simulink model "FunctionalArchitectureProj"  (R2023b)
settings: Solver=VariableStepAuto  StartTime=0.0  StopTime=10.0  RelTol=1e-3
(part 1 of 3)
settings Model: Creator=carol  LastModifiedBy=carol

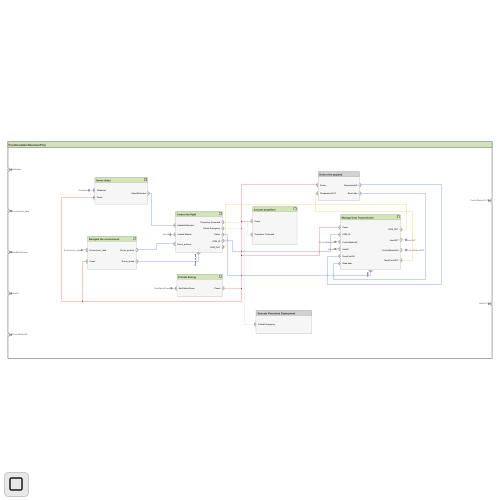
[thumbnail: Simulink's stored preview of the top-level diagram]
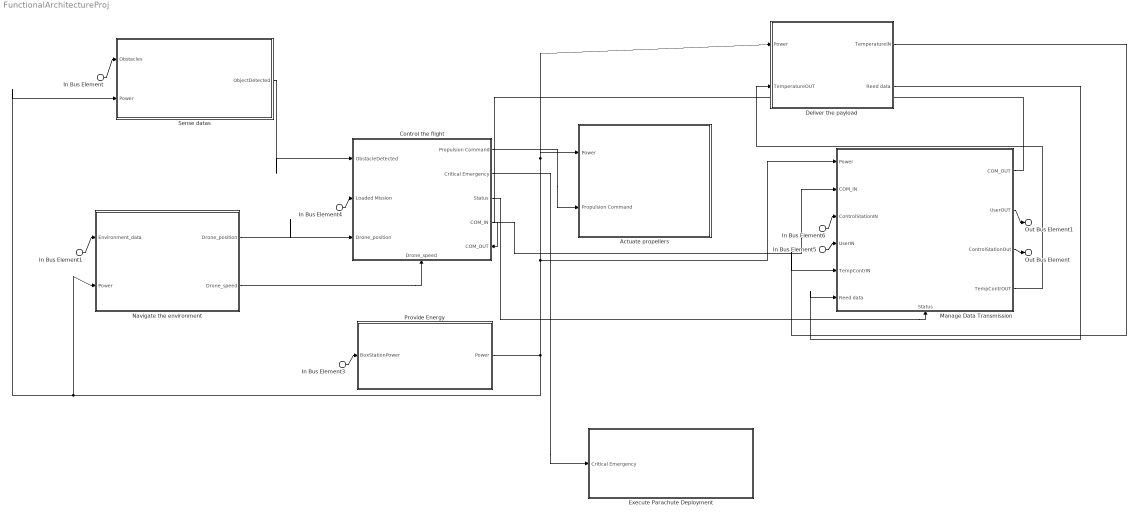
== system FunctionalArchitectureProj ==
  In Bus Element : Inport  PortName=Obstacles
  In Bus Element1 : Inport  Port=2  PortName=Environment_data
  In Bus Element3 : Inport  Port=3  PortName=BoxStationPower
  In Bus Element4 : Inport  Port=4  PortName=UserIN
  In Bus Element5 : Inport  Port=4  PortName=UserIN
  In Bus Element6 : Inport  Port=5  PortName=ControlStationIN
  " Execute Parachute Deployment" : Subsystem
      settings: PortSchema="{\"entries\":[{\"content\":{\"headerSize\":26,\"margin\":15,\"minimumSpacing\":25,\"sides\":[{\"content\":{\"connectorIds\":[\"In1\"]},\"type\":\"ConnectorPlacement.EquallySpacedRectSide\",\"uuid\":\"8049ad02-19ac-4f14-9b36-a42a8615a652\"},{\"content\":{\"side\":\"RIGHT\"},\"type\":\"ConnectorPlacement.EquallySpacedRectSide\",\"uuid\":\"a3e2e02d-3567-418c-afac-b08313eb92f4\"},{\"content\":{\"side\":\"TOP\"},\"type\":\"ConnectorPlacement.EquallySpacedRectSide\",\"uuid\":\"0a99e400-62af-4ce6-9b2a-3ec4b8645f60\"},{\"content\":{\"side\":\"BOTTOM\"},\"type\":\"ConnectorPlacement.EquallySpacedRectSide\",\"uuid\":\"e83c7a6e-944d-4583-b49e-8615a84d262f\"}]},\"type\":\"ConnectorPlacement.EquallySpacedConnector\",\"uuid\":\"ada0285e-d286-47a3-bd64-ce4f3c6c3017\"}],\"packageUris\":[\"http://schema.mathworks.com/mf0/Connector/R2020b\"],\"version\":\"1.0\"}"
  Actuate propellers : Subsystem
      settings: PortSchema="{\"entries\":[{\"content\":{\"headerSize\":26,\"margin\":15,\"minimumSpacing\":25,\"sides\":[{\"content\":{\"connectorIds\":[\"In1\",\"In2\"]},\"type\":\"ConnectorPlacement.EquallySpacedRectSide\",\"uuid\":\"9cca9539-0a36-4124-b22c-ee31f3591a67\"},{\"content\":{\"side\":\"RIGHT\"},\"type\":\"ConnectorPlacement.EquallySpacedRectSide\",\"uuid\":\"eebe1ec1-c849-468b-8863-53f0cc841d23\"},{\"content\":{\"side\":\"TOP\"},\"type\":\"ConnectorPlacement.EquallySpacedRectSide\",\"uuid\":\"8f1c4dda-9d7f-4fb5-99d0-4e96ed432329\"}]},\"type\":\"ConnectorPlacement.EquallySpacedConnector\",\"uuid\":\"f7d57f3a-667c-4dfa-8f30-8433699dfbc6\"}],\"packageUris\":[\"http://schema.mathworks.com/mf0/Connector/R2020b\"],\"version\":\"1.0\"}"
  Control the flight : Subsystem
      settings: PortSchema="{\"entries\":[{\"content\":{\"headerSize\":26,\"margin\":15,\"minimumSpacing\":25,\"sides\":[{\"content\":{\"connectorIds\":[\"In3\",\"In4\",\"In5\"]},\"type\":\"ConnectorPlacement.EquallySpacedRectSide\",\"uuid\":\"6ae6270c-bff4-4a0d-8fba-8fdec87b0a05\"},{\"content\":{\"connectorIds\":[\"Out1\",\"Out2\",\"Out3\",\"Out4\",\"In1\"],\"side\":\"RIGHT\"},\"type\":\"ConnectorPlacement.EquallySpacedRectSide\",\"uuid\":\"f3a0045b-bb3b-40f9-afd5-e1537ff3eeca\"},{\"content\":{\"side\":\"TOP\"},\"type\":\"ConnectorPlacement.EquallySpacedRectSide\",\"uuid\":\"e89a58f2-90b0-468c-bb6a-95617af68e24\"},{\"content\":{\"connectorIds\":[\"In2\"],\"side\":\"BOTTOM\"},\"type\":\"ConnectorPlacement.EquallySpacedRectSide\",\"uuid\":\"5f2fc7ae-0fcb-4b02-9512-f183f1206c8f\"}]},\"type\":\"ConnectorPlacement.EquallySpacedConnector\",\"uuid\":\"066eb43c-7b96-4660-9f29-628dd77a5b3b\"}],\"packageUris\":[\"http://schema.mathworks.com/mf0/Connector/R2020b\"],\"version\":\"1.0\"}"
  Deliver the payload : Subsystem
      settings: PortSchema="{\"entries\":[{\"content\":{\"headerSize\":26,\"margin\":15,\"minimumSpacing\":25,\"sides\":[{\"content\":{\"connectorIds\":[\"In1\",\"In2\"]},\"type\":\"ConnectorPlacement.EquallySpacedRectSide\",\"uuid\":\"8049ad02-19ac-4f14-9b36-a42a8615a652\"},{\"content\":{\"connectorIds\":[\"Out2\",\"Out1\"],\"side\":\"RIGHT\"},\"type\":\"ConnectorPlacement.EquallySpacedRectSide\",\"uuid\":\"a3e2e02d-3567-418c-afac-b08313eb92f4\"},{\"content\":{\"side\":\"TOP\"},\"type\":\"ConnectorPlacement.EquallySpacedRectSide\",\"uuid\":\"0a99e400-62af-4ce6-9b2a-3ec4b8645f60\"}]},\"type\":\"ConnectorPlacement.EquallySpacedConnector\",\"uuid\":\"ada0285e-d286-47a3-bd64-ce4f3c6c3017\"}],\"packageUris\":[\"http://schema.mathworks.com/mf0/Connector/R2020b\"],\"version\":\"1.0\"}"
  "Manage Data Transmission " : Subsystem
      settings: PortSchema="{\"entries\":[{\"content\":{\"headerSize\":26,\"margin\":15,\"minimumSpacing\":25,\"sides\":[{\"content\":{\"connectorIds\":[\"In2\",\"In3\",\"In4\",\"In5\",\"In7\",\"In6\"]},\"type\":\"ConnectorPlacement.EquallySpacedRectSide\",\"uuid\":\"9c17b9ef-2834-4c82-b9e5-e6d3fc257de6\"},{\"content\":{\"connectorIds\":[\"Out1\",\"Out2\",\"Out3\",\"Out4\"],\"side\":\"RIGHT\"},\"type\":\"ConnectorPlacement.EquallySpacedRectSide\",\"uuid\":\"9ecb8183-c057-4821-b5b4-2d9c431b5fb2\"},{\"content\":{\"side\":\"TOP\"},\"type\":\"ConnectorPlacement.EquallySpacedRectSide\",\"uuid\":\"bcbced7c-61ac-4e5d-8c11-0c5bb0f95d66\"},{\"content\":{\"connectorIds\":[\"In1\"],\"side\":\"BOTTOM\"},\"type\":\"ConnectorPlacement.EquallySpacedRectSide\",\"uuid\":\"08cd3b33-b135-4af9-aec5-206e0f2419c0\"}]},\"type\":\"ConnectorPlacement.EquallySpacedConnector\",\"uuid\":\"9e4a88fc-7b2c-4c70-8e8f-1bc090782de6\"}],\"packageUris\":[\"http://schema.mathworks.com/mf0/Connector/R2020b\"],\"version\":\"1.0\"}"
  Navigate the environment : Subsystem
      settings: PortSchema="{\"entries\":[{\"content\":{\"headerSize\":26,\"margin\":15,\"minimumSpacing\":25,\"sides\":[{\"content\":{\"connectorIds\":[\"In1\",\"In2\"]},\"type\":\"ConnectorPlacement.EquallySpacedRectSide\",\"uuid\":\"3b5ec35b-efef-42bc-989f-0358b373f88c\"},{\"content\":{\"connectorIds\":[\"Out1\",\"Out2\"],\"side\":\"RIGHT\"},\"type\":\"ConnectorPlacement.EquallySpacedRectSide\",\"uuid\":\"39a24d49-19b9-4508-91cd-8aceba2ac1ea\"},{\"content\":{\"side\":\"TOP\"},\"type\":\"ConnectorPlacement.EquallySpacedRectSide\",\"uuid\":\"1edcc8ed-84b2-4c5f-810f-53183898c4f5\"}]},\"type\":\"ConnectorPlacement.EquallySpacedConnector\",\"uuid\":\"9d581d8a-2dea-49e6-903e-7a6990d5505f\"}],\"packageUris\":[\"http://schema.mathworks.com/mf0/Connector/R2020b\"],\"version\":\"1.0\"}"
  Provide Energy : Subsystem
      settings: PortSchema="{\"entries\":[{\"content\":{\"headerSize\":26,\"margin\":15,\"minimumSpacing\":25,\"sides\":[{\"content\":{\"connectorIds\":[\"In1\"]},\"type\":\"ConnectorPlacement.EquallySpacedRectSide\",\"uuid\":\"6ae6270c-bff4-4a0d-8fba-8fdec87b0a05\"},{\"content\":{\"connectorIds\":[\"Out1\"],\"side\":\"RIGHT\"},\"type\":\"ConnectorPlacement.EquallySpacedRectSide\",\"uuid\":\"f3a0045b-bb3b-40f9-afd5-e1537ff3eeca\"},{\"content\":{\"side\":\"TOP\"},\"type\":\"ConnectorPlacement.EquallySpacedRectSide\",\"uuid\":\"e89a58f2-90b0-468c-bb6a-95617af68e24\"}]},\"type\":\"ConnectorPlacement.EquallySpacedConnector\",\"uuid\":\"066eb43c-7b96-4660-9f29-628dd77a5b3b\"}],\"packageUris\":[\"http://schema.mathworks.com/mf0/Connector/R2020b\"],\"version\":\"1.0\"}"
  Sense datas : Subsystem
      settings: PortSchema="{\"entries\":[{\"content\":{\"headerSize\":26,\"margin\":15,\"minimumSpacing\":25,\"sides\":[{\"content\":{\"connectorIds\":[\"In1\",\"In2\"]},\"type\":\"ConnectorPlacement.EquallySpacedRectSide\",\"uuid\":\"6ae6270c-bff4-4a0d-8fba-8fdec87b0a05\"},{\"content\":{\"connectorIds\":[\"Out1\"],\"side\":\"RIGHT\"},\"type\":\"ConnectorPlacement.EquallySpacedRectSide\",\"uuid\":\"f3a0045b-bb3b-40f9-afd5-e1537ff3eeca\"},{\"content\":{\"side\":\"TOP\"},\"type\":\"ConnectorPlacement.EquallySpacedRectSide\",\"uuid\":\"e89a58f2-90b0-468c-bb6a-95617af68e24\"}]},\"type\":\"ConnectorPlacement.EquallySpacedConnector\",\"uuid\":\"066eb43c-7b96-4660-9f29-628dd77a5b3b\"}],\"packageUris\":[\"http://schema.mathworks.com/mf0/Connector/R2020b\"],\"version\":\"1.0\"}"
  Out Bus Element : Outport  PortName=ControlStationOUT
  Out Bus Element1 : Outport  Port=2  PortName=UserOUT
  wires:
  In Bus Element3/1 -> Provide Energy/1(BoxStationPower)
  In Bus Element1/1 -> Navigate the environment/1(Environment_data)
  In Bus Element/1 -> Sense datas/1(Obstacles)
  Control the flight/1(Propulsion Command) -> Actuate propellers/2(Propulsion Command)
  Sense datas/1(ObjectDetected) -> Control the flight/3(ObstacleDetected)
  Navigate the environment/1(Drone_position) -> Control the flight/5(Drone_position)
  Navigate the environment/2(Drone_speed) -> Control the flight/2(Drone_speed)
  Provide Energy/1(Power) -> Navigate the environment/2(Power), Sense datas/2(Power), "Manage Data Transmission "/2(Power), Deliver the payload/1(Power), Actuate propellers/1(Power)
  Control the flight/2(Critical Emergency) -> " Execute Parachute Deployment"/1(Critical Emergency)
  Control the flight/3(Status) -> "Manage Data Transmission "/1(Status)
  Control the flight/4(COM_IN) -> "Manage Data Transmission "/3(COM_IN)
  "Manage Data Transmission "/1(COM_OUT) -> Control the flight/1(COM_OUT)
  In Bus Element4/1 -> Control the flight/4(Loaded Mission)
  In Bus Element5/1 -> "Manage Data Transmission "/5(UserIN)
  "Manage Data Transmission "/2(UserOUT) -> Out Bus Element1/1
  "Manage Data Transmission "/3(ControlStationOut) -> Out Bus Element/1
  "Manage Data Transmission "/4(TempContrOUT) -> Deliver the payload/2(TemperatureOUT)
  Deliver the payload/2(TemperatureIN) -> "Manage Data Transmission "/7(TempContrIN)
  Deliver the payload/1(Reed data) -> "Manage Data Transmission "/6(Reed data)
  In Bus Element6/1 -> "Manage Data Transmission "/4(ControlStationIN)

== system FunctionalArchitectureProj/ Execute Parachute Deployment ==
  Bus Element In1 : Inport  PortName=Critical Emergency
  Detect emergency : Subsystem
      settings: PortSchema="{\"entries\":[{\"content\":{\"headerSize\":26,\"margin\":15,\"minimumSpacing\":25,\"sides\":[{\"content\":{\"connectorIds\":[\"In1\"]},\"type\":\"ConnectorPlacement.EquallySpacedRectSide\",\"uuid\":\"8049ad02-19ac-4f14-9b36-a42a8615a652\"},{\"content\":{\"connectorIds\":[\"Out1\"],\"side\":\"RIGHT\"},\"type\":\"ConnectorPlacement.EquallySpacedRectSide\",\"uuid\":\"a3e2e02d-3567-418c-afac-b08313eb92f4\"},{\"content\":{\"side\":\"TOP\"},\"type\":\"ConnectorPlacement.EquallySpacedRectSide\",\"uuid\":\"0a99e400-62af-4ce6-9b2a-3ec4b8645f60\"}]},\"type\":\"ConnectorPlacement.EquallySpacedConnector\",\"uuid\":\"ada0285e-d286-47a3-bd64-ce4f3c6c3017\"}],\"packageUris\":[\"http://schema.mathworks.com/mf0/Connector/R2020b\"],\"version\":\"1.0\"}"
  Execute the parachute : Subsystem
      settings: PortSchema="{\"entries\":[{\"content\":{\"headerSize\":26,\"margin\":15,\"minimumSpacing\":25,\"sides\":[{\"content\":{\"connectorIds\":[\"In1\"]},\"type\":\"ConnectorPlacement.EquallySpacedRectSide\",\"uuid\":\"8049ad02-19ac-4f14-9b36-a42a8615a652\"},{\"content\":{\"side\":\"RIGHT\"},\"type\":\"ConnectorPlacement.EquallySpacedRectSide\",\"uuid\":\"a3e2e02d-3567-418c-afac-b08313eb92f4\"},{\"content\":{\"side\":\"TOP\"},\"type\":\"ConnectorPlacement.EquallySpacedRectSide\",\"uuid\":\"0a99e400-62af-4ce6-9b2a-3ec4b8645f60\"}]},\"type\":\"ConnectorPlacement.EquallySpacedConnector\",\"uuid\":\"ada0285e-d286-47a3-bd64-ce4f3c6c3017\"}],\"packageUris\":[\"http://schema.mathworks.com/mf0/Connector/R2020b\"],\"version\":\"1.0\"}"
  Trigger the mechanism : Subsystem
      settings: PortSchema="{\"entries\":[{\"content\":{\"headerSize\":26,\"margin\":15,\"minimumSpacing\":25,\"sides\":[{\"content\":{\"connectorIds\":[\"In1\"]},\"type\":\"ConnectorPlacement.EquallySpacedRectSide\",\"uuid\":\"8049ad02-19ac-4f14-9b36-a42a8615a652\"},{\"content\":{\"connectorIds\":[\"Out1\"],\"side\":\"RIGHT\"},\"type\":\"ConnectorPlacement.EquallySpacedRectSide\",\"uuid\":\"a3e2e02d-3567-418c-afac-b08313eb92f4\"},{\"content\":{\"side\":\"TOP\"},\"type\":\"ConnectorPlacement.EquallySpacedRectSide\",\"uuid\":\"0a99e400-62af-4ce6-9b2a-3ec4b8645f60\"}]},\"type\":\"ConnectorPlacement.EquallySpacedConnector\",\"uuid\":\"ada0285e-d286-47a3-bd64-ce4f3c6c3017\"}],\"packageUris\":[\"http://schema.mathworks.com/mf0/Connector/R2020b\"],\"version\":\"1.0\"}"
  wires:
  Detect emergency/1(alert_signal) -> Trigger the mechanism/1(alert_signal)
  Trigger the mechanism/1(Trigger _signal) -> Execute the parachute/1(Trigger _signal)
  Bus Element In1/1 -> Detect emergency/1(Critical Emergency)

== system FunctionalArchitectureProj/Actuate propellers ==
  Bus Element In1 : Inport  PortName=Power
  Bus Element In6 : Inport  Port=2  PortName=Propulsion Command
  Regulate speed of Propeller : Subsystem
      settings: PortSchema="{\"entries\":[{\"content\":{\"headerSize\":26,\"margin\":15,\"minimumSpacing\":25,\"sides\":[{\"content\":{\"connectorIds\":[\"In2\"]},\"type\":\"ConnectorPlacement.EquallySpacedRectSide\",\"uuid\":\"c0b5e0bb-d2bf-4d40-b1ad-0d63f5f2311e\"},{\"content\":{\"connectorIds\":[\"Out1\"],\"side\":\"RIGHT\"},\"type\":\"ConnectorPlacement.EquallySpacedRectSide\",\"uuid\":\"73104a81-7012-49ca-8030-68cbb7243dfa\"},{\"content\":{\"side\":\"TOP\"},\"type\":\"ConnectorPlacement.EquallySpacedRectSide\",\"uuid\":\"7c311739-eaa1-403c-a576-4458554363b2\"},{\"content\":{\"connectorIds\":[\"In1\"],\"side\":\"BOTTOM\"},\"type\":\"ConnectorPlacement.EquallySpacedRectSide\",\"uuid\":\"afa3ef7d-980f-4119-97e5-3dc0677e5f7e\"}]},\"type\":\"ConnectorPlacement.EquallySpacedConnector\",\"uuid\":\"83a80a93-0958-4176-98e5-b02d609066aa\"}],\"packageUris\":[\"http://schema.mathworks.com/mf0/Connector/R2020b\"],\"version\":\"1.0\"}"
  Set Target speed of propellers : Subsystem
      settings: PortSchema="{\"entries\":[{\"content\":{\"headerSize\":26,\"margin\":15,\"minimumSpacing\":25,\"sides\":[{\"content\":{\"connectorIds\":[\"In1\"]},\"type\":\"ConnectorPlacement.EquallySpacedRectSide\",\"uuid\":\"c0b5e0bb-d2bf-4d40-b1ad-0d63f5f2311e\"},{\"content\":{\"connectorIds\":[\"Out1\"],\"side\":\"RIGHT\"},\"type\":\"ConnectorPlacement.EquallySpacedRectSide\",\"uuid\":\"73104a81-7012-49ca-8030-68cbb7243dfa\"},{\"content\":{\"side\":\"TOP\"},\"type\":\"ConnectorPlacement.EquallySpacedRectSide\",\"uuid\":\"7c311739-eaa1-403c-a576-4458554363b2\"}]},\"type\":\"ConnectorPlacement.EquallySpacedConnector\",\"uuid\":\"83a80a93-0958-4176-98e5-b02d609066aa\"}],\"packageUris\":[\"http://schema.mathworks.com/mf0/Connector/R2020b\"],\"version\":\"1.0\"}"
  Split the energy : Subsystem
      settings: PortSchema="{\"entries\":[{\"content\":{\"headerSize\":26,\"margin\":15,\"minimumSpacing\":25,\"sides\":[{\"content\":{\"connectorIds\":[\"In1\",\"In2\"]},\"type\":\"ConnectorPlacement.EquallySpacedRectSide\",\"uuid\":\"c0b5e0bb-d2bf-4d40-b1ad-0d63f5f2311e\"},{\"content\":{\"connectorIds\":[\"Out1\"],\"side\":\"RIGHT\"},\"type\":\"ConnectorPlacement.EquallySpacedRectSide\",\"uuid\":\"73104a81-7012-49ca-8030-68cbb7243dfa\"},{\"content\":{\"connectorIds\":[],\"side\":\"TOP\"},\"type\":\"ConnectorPlacement.EquallySpacedRectSide\",\"uuid\":\"7c311739-eaa1-403c-a576-4458554363b2\"},{\"content\":{\"connectorIds\":[],\"side\":\"BOTTOM\"},\"type\":\"ConnectorPlacement.EquallySpacedRectSide\",\"uuid\":\"ef70e0e5-7c28-4d60-a2ab-1af0db1b5348\"}]},\"type\":\"ConnectorPlacement.EquallySpacedConnector\",\"uuid\":\"83a80a93-0958-4176-98e5-b02d609066aa\"}],\"packageUris\":[\"http://schema.mathworks.com/mf0/Connector/R2020b\"],\"version\":\"1.0\"}"
  wires:
  Bus Element In6/1 -> Set Target speed of propellers/1(Propulsion Command)
  Set Target speed of propellers/1(Target_Speed) -> Regulate speed of Propeller/2(Target_Speed)
  Regulate speed of Propeller/1(data) -> Split the energy/2(data)
  Split the energy/1(Single Motor Voltage) -> Regulate speed of Propeller/1(Single Motor Voltage)
  Bus Element In1/1 -> Split the energy/1(Power)

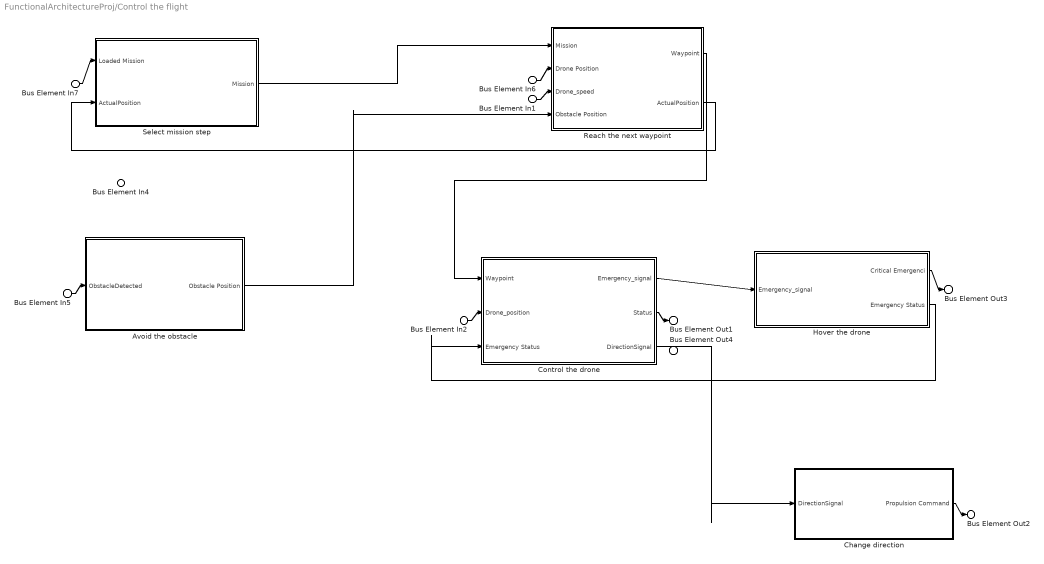
== system FunctionalArchitectureProj/Control the flight ==
  Bus Element In4 : Inport  PortName=COM_OUT
  Bus Element In1 : Inport  Port=2  PortName=Drone_speed
  Bus Element In5 : Inport  Port=3  PortName=ObstacleDetected
  Bus Element In7 : Inport  Port=4  PortName=Loaded Mission
  Bus Element In6 : Inport  Port=5  PortName=Drone_position
  Bus Element In2 : Inport  Port=5  PortName=Drone_position
  Avoid the obstacle : Subsystem
      settings: PortSchema="{\"entries\":[{\"content\":{\"headerSize\":26,\"margin\":15,\"minimumSpacing\":25,\"sides\":[{\"content\":{\"connectorIds\":[\"In1\"]},\"type\":\"ConnectorPlacement.EquallySpacedRectSide\",\"uuid\":\"9cca9539-0a36-4124-b22c-ee31f3591a67\"},{\"content\":{\"connectorIds\":[\"Out1\"],\"side\":\"RIGHT\"},\"type\":\"ConnectorPlacement.EquallySpacedRectSide\",\"uuid\":\"eebe1ec1-c849-468b-8863-53f0cc841d23\"},{\"content\":{\"connectorIds\":[],\"side\":\"TOP\"},\"type\":\"ConnectorPlacement.EquallySpacedRectSide\",\"uuid\":\"8f1c4dda-9d7f-4fb5-99d0-4e96ed432329\"}]},\"type\":\"ConnectorPlacement.EquallySpacedConnector\",\"uuid\":\"f7d57f3a-667c-4dfa-8f30-8433699dfbc6\"}],\"packageUris\":[\"http://schema.mathworks.com/mf0/Connector/R2020b\"],\"version\":\"1.0\"}"
  Change direction : Subsystem
      settings: PortSchema="{\"entries\":[{\"content\":{\"headerSize\":26,\"margin\":15,\"minimumSpacing\":25,\"sides\":[{\"content\":{\"connectorIds\":[\"In1\"]},\"type\":\"ConnectorPlacement.EquallySpacedRectSide\",\"uuid\":\"9cca9539-0a36-4124-b22c-ee31f3591a67\"},{\"content\":{\"connectorIds\":[\"Out1\"],\"side\":\"RIGHT\"},\"type\":\"ConnectorPlacement.EquallySpacedRectSide\",\"uuid\":\"eebe1ec1-c849-468b-8863-53f0cc841d23\"},{\"content\":{\"side\":\"TOP\"},\"type\":\"ConnectorPlacement.EquallySpacedRectSide\",\"uuid\":\"8f1c4dda-9d7f-4fb5-99d0-4e96ed432329\"}]},\"type\":\"ConnectorPlacement.EquallySpacedConnector\",\"uuid\":\"f7d57f3a-667c-4dfa-8f30-8433699dfbc6\"}],\"packageUris\":[\"http://schema.mathworks.com/mf0/Connector/R2020b\"],\"version\":\"1.0\"}"
  Control the drone : Subsystem
      settings: PortSchema="{\"entries\":[{\"content\":{\"headerSize\":26,\"margin\":15,\"minimumSpacing\":25,\"sides\":[{\"content\":{\"connectorIds\":[\"In1\",\"In2\",\"In3\"]},\"type\":\"ConnectorPlacement.EquallySpacedRectSide\",\"uuid\":\"ae43e0f9-cb81-4c7d-a5a1-6ddd261c3f36\"},{\"content\":{\"connectorIds\":[\"Out1\",\"Out2\",\"Out3\"],\"side\":\"RIGHT\"},\"type\":\"ConnectorPlacement.EquallySpacedRectSide\",\"uuid\":\"454013ea-826f-4879-bd33-a0fc10a3e69e\"},{\"content\":{\"connectorIds\":[],\"side\":\"TOP\"},\"type\":\"ConnectorPlacement.EquallySpacedRectSide\",\"uuid\":\"d045879a-9dfe-4c38-a274-6118b00e003b\"}]},\"type\":\"ConnectorPlacement.EquallySpacedConnector\",\"uuid\":\"e33c714e-0ae2-4a56-8ce0-f9b8de85daa2\"}],\"packageUris\":[\"http://schema.mathworks.com/mf0/Connector/R2020b\"],\"version\":\"1.0\"}"
  Hover the drone : Subsystem
      settings: PortSchema="{\"entries\":[{\"content\":{\"headerSize\":26,\"margin\":15,\"minimumSpacing\":25,\"sides\":[{\"content\":{\"connectorIds\":[\"In1\"]},\"type\":\"ConnectorPlacement.EquallySpacedRectSide\",\"uuid\":\"ae43e0f9-cb81-4c7d-a5a1-6ddd261c3f36\"},{\"content\":{\"connectorIds\":[\"Out1\",\"Out2\"],\"side\":\"RIGHT\"},\"type\":\"ConnectorPlacement.EquallySpacedRectSide\",\"uuid\":\"454013ea-826f-4879-bd33-a0fc10a3e69e\"},{\"content\":{\"connectorIds\":[],\"side\":\"TOP\"},\"type\":\"ConnectorPlacement.EquallySpacedRectSide\",\"uuid\":\"d045879a-9dfe-4c38-a274-6118b00e003b\"}]},\"type\":\"ConnectorPlacement.EquallySpacedConnector\",\"uuid\":\"e33c714e-0ae2-4a56-8ce0-f9b8de85daa2\"}],\"packageUris\":[\"http://schema.mathworks.com/mf0/Connector/R2020b\"],\"version\":\"1.0\"}"
  Reach the next waypoint : Subsystem
      settings: PortSchema="{\"entries\":[{\"content\":{\"headerSize\":26,\"margin\":15,\"minimumSpacing\":25,\"sides\":[{\"content\":{\"connectorIds\":[\"In1\",\"In2\",\"In3\",\"In4\"]},\"type\":\"ConnectorPlacement.EquallySpacedRectSide\",\"uuid\":\"ae43e0f9-cb81-4c7d-a5a1-6ddd261c3f36\"},{\"content\":{\"connectorIds\":[\"Out2\",\"Out1\"],\"side\":\"RIGHT\"},\"type\":\"ConnectorPlacement.EquallySpacedRectSide\",\"uuid\":\"454013ea-826f-4879-bd33-a0fc10a3e69e\"},{\"content\":{\"connectorIds\":[],\"side\":\"TOP\"},\"type\":\"ConnectorPlacement.EquallySpacedRectSide\",\"uuid\":\"d045879a-9dfe-4c38-a274-6118b00e003b\"}]},\"type\":\"ConnectorPlacement.EquallySpacedConnector\",\"uuid\":\"e33c714e-0ae2-4a56-8ce0-f9b8de85daa2\"}],\"packageUris\":[\"http://schema.mathworks.com/mf0/Connector/R2020b\"],\"version\":\"1.0\"}"
  Select mission step : Subsystem
      settings: PortSchema="{\"entries\":[{\"content\":{\"headerSize\":26,\"margin\":15,\"minimumSpacing\":25,\"sides\":[{\"content\":{\"connectorIds\":[\"In1\",\"In2\"]},\"type\":\"ConnectorPlacement.EquallySpacedRectSide\",\"uuid\":\"ae43e0f9-cb81-4c7d-a5a1-6ddd261c3f36\"},{\"content\":{\"connectorIds\":[\"Out1\"],\"side\":\"RIGHT\"},\"type\":\"ConnectorPlacement.EquallySpacedRectSide\",\"uuid\":\"454013ea-826f-4879-bd33-a0fc10a3e69e\"},{\"content\":{\"connectorIds\":[],\"side\":\"TOP\"},\"type\":\"ConnectorPlacement.EquallySpacedRectSide\",\"uuid\":\"d045879a-9dfe-4c38-a274-6118b00e003b\"}]},\"type\":\"ConnectorPlacement.EquallySpacedConnector\",\"uuid\":\"e33c714e-0ae2-4a56-8ce0-f9b8de85daa2\"}],\"packageUris\":[\"http://schema.mathworks.com/mf0/Connector/R2020b\"],\"version\":\"1.0\"}"
  Bus Element Out2 : Outport  PortName=Propulsion Command
  Bus Element Out3 : Outport  Port=2  PortName=Critical Emergency
  Bus Element Out1 : Outport  Port=3  PortName=Status
  Bus Element Out4 : Outport  Port=4  PortName=COM_IN
  wires:
  Bus Element In5/1 -> Avoid the obstacle/1(ObstacleDetected)
  Bus Element In6/1 -> Reach the next waypoint/2(Drone Position)
  Select mission step/1(Mission) -> Reach the next waypoint/1(Mission)
  Reach the next waypoint/1(ActualPosition) -> Select mission step/2(ActualPosition)
  Bus Element In7/1 -> Select mission step/1(Loaded Mission)
  Change direction/1(Propulsion Command) -> Bus Element Out2/1
  Bus Element In1/1 -> Reach the next waypoint/3(Drone_speed)
  Control the drone/2(Status) -> Bus Element Out1/1
  Avoid the obstacle/1(Obstacle Position) -> Reach the next waypoint/4(Obstacle Position)
  Reach the next waypoint/2(Waypoint) -> Control the drone/1(Waypoint)
  Control the drone/3(DirectionSignal) -> Change direction/1(DirectionSignal)
  Bus Element In2/1 -> Control the drone/2(Drone_position)
  Control the drone/1(Emergency_signal) -> Hover the drone/1(Emergency_signal)
  Hover the drone/1(Critical Emergenci) -> Bus Element Out3/1
  Hover the drone/2(Emergency Status) -> Control the drone/3(Emergency Status)

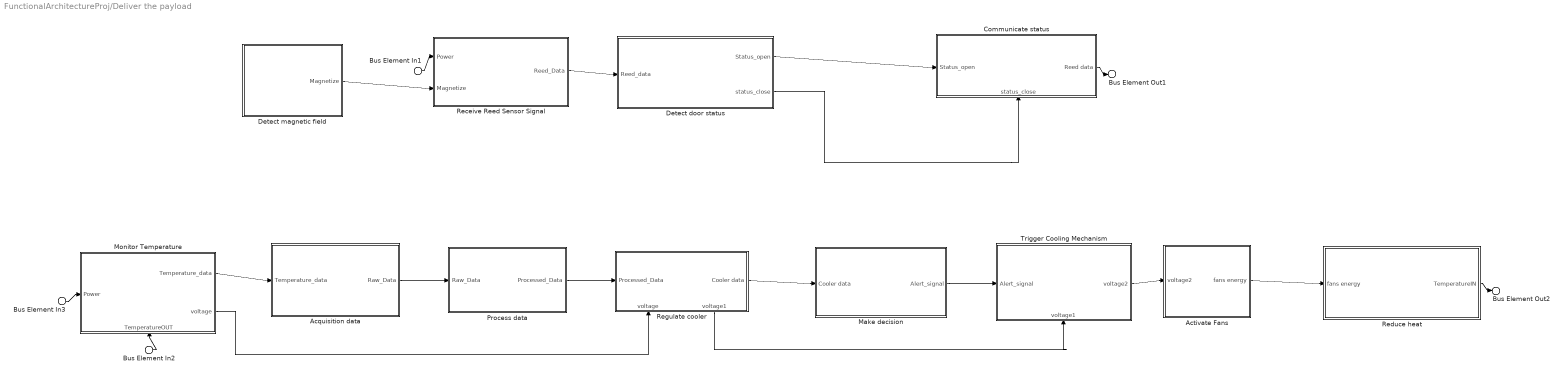
== system FunctionalArchitectureProj/Deliver the payload ==
  Bus Element In1 : Inport  PortName=Power
  Bus Element In3 : Inport  PortName=Power
  Bus Element In2 : Inport  Port=2  PortName=TemperatureOUT
  Acquisition data : Subsystem
      settings: PortSchema="{\"entries\":[{\"content\":{\"headerSize\":26,\"margin\":15,\"minimumSpacing\":25,\"sides\":[{\"content\":{\"connectorIds\":[\"In1\"]},\"type\":\"ConnectorPlacement.EquallySpacedRectSide\",\"uuid\":\"8049ad02-19ac-4f14-9b36-a42a8615a652\"},{\"content\":{\"connectorIds\":[\"Out1\"],\"side\":\"RIGHT\"},\"type\":\"ConnectorPlacement.EquallySpacedRectSide\",\"uuid\":\"a3e2e02d-3567-418c-afac-b08313eb92f4\"},{\"content\":{\"side\":\"TOP\"},\"type\":\"ConnectorPlacement.EquallySpacedRectSide\",\"uuid\":\"0a99e400-62af-4ce6-9b2a-3ec4b8645f60\"}]},\"type\":\"ConnectorPlacement.EquallySpacedConnector\",\"uuid\":\"ada0285e-d286-47a3-bd64-ce4f3c6c3017\"}],\"packageUris\":[\"http://schema.mathworks.com/mf0/Connector/R2020b\"],\"version\":\"1.0\"}"
  Activate Fans : Subsystem
      settings: PortSchema="{\"entries\":[{\"content\":{\"headerSize\":26,\"margin\":15,\"minimumSpacing\":25,\"sides\":[{\"content\":{\"connectorIds\":[\"In1\"]},\"type\":\"ConnectorPlacement.EquallySpacedRectSide\",\"uuid\":\"54e1fb7b-9e45-462f-884a-02984b69df8e\"},{\"content\":{\"connectorIds\":[\"Out1\"],\"side\":\"RIGHT\"},\"type\":\"ConnectorPlacement.EquallySpacedRectSide\",\"uuid\":\"bc959cb6-5763-4613-9c0f-216dfc1c8721\"},{\"content\":{\"side\":\"TOP\"},\"type\":\"ConnectorPlacement.EquallySpacedRectSide\",\"uuid\":\"3094b2e1-2656-4eb0-a370-e33613cb9a3e\"}]},\"type\":\"ConnectorPlacement.EquallySpacedConnector\",\"uuid\":\"4e036095-9cf9-4f63-b3c0-cf00d09848ce\"}],\"packageUris\":[\"http://schema.mathworks.com/mf0/Connector/R2020b\"],\"version\":\"1.0\"}"
  Communicate status : Subsystem
      settings: PortSchema="{\"entries\":[{\"content\":{\"headerSize\":26,\"margin\":15,\"minimumSpacing\":25,\"sides\":[{\"content\":{\"connectorIds\":[\"In1\"]},\"type\":\"ConnectorPlacement.EquallySpacedRectSide\",\"uuid\":\"8049ad02-19ac-4f14-9b36-a42a8615a652\"},{\"content\":{\"connectorIds\":[\"Out1\"],\"side\":\"RIGHT\"},\"type\":\"ConnectorPlacement.EquallySpacedRectSide\",\"uuid\":\"a3e2e02d-3567-418c-afac-b08313eb92f4\"},{\"content\":{\"side\":\"TOP\"},\"type\":\"ConnectorPlacement.EquallySpacedRectSide\",\"uuid\":\"0a99e400-62af-4ce6-9b2a-3ec4b8645f60\"},{\"content\":{\"connectorIds\":[\"In2\"],\"side\":\"BOTTOM\"},\"type\":\"ConnectorPlacement.EquallySpacedRectSide\",\"uuid\":\"af5b728c-4ca3-4e93-bc61-3fa3a4a27f8e\"}]},\"type\":\"ConnectorPlacement.EquallySpacedConnector\",\"uuid\":\"ada0285e-d286-47a3-bd64-ce4f3c6c3017\"}],\"packageUris\":[\"http://schema.mathworks.com/mf0/Connector/R2020b\"],\"version\":\"1.0\"}"
  Detect door status : Subsystem
      settings: PortSchema="{\"entries\":[{\"content\":{\"headerSize\":26,\"margin\":15,\"minimumSpacing\":25,\"sides\":[{\"content\":{\"connectorIds\":[\"In1\"]},\"type\":\"ConnectorPlacement.EquallySpacedRectSide\",\"uuid\":\"8049ad02-19ac-4f14-9b36-a42a8615a652\"},{\"content\":{\"connectorIds\":[\"Out1\",\"Out2\"],\"side\":\"RIGHT\"},\"type\":\"ConnectorPlacement.EquallySpacedRectSide\",\"uuid\":\"a3e2e02d-3567-418c-afac-b08313eb92f4\"},{\"content\":{\"side\":\"TOP\"},\"type\":\"ConnectorPlacement.EquallySpacedRectSide\",\"uuid\":\"0a99e400-62af-4ce6-9b2a-3ec4b8645f60\"}]},\"type\":\"ConnectorPlacement.EquallySpacedConnector\",\"uuid\":\"ada0285e-d286-47a3-bd64-ce4f3c6c3017\"}],\"packageUris\":[\"http://schema.mathworks.com/mf0/Connector/R2020b\"],\"version\":\"1.0\"}"
  Detect magnetic field : Subsystem
      settings: PortSchema="{\"entries\":[{\"content\":{\"headerSize\":26,\"margin\":15,\"minimumSpacing\":25,\"sides\":[{\"content\":{},\"type\":\"ConnectorPlacement.EquallySpacedRectSide\",\"uuid\":\"8049ad02-19ac-4f14-9b36-a42a8615a652\"},{\"content\":{\"connectorIds\":[\"Out1\"],\"side\":\"RIGHT\"},\"type\":\"ConnectorPlacement.EquallySpacedRectSide\",\"uuid\":\"a3e2e02d-3567-418c-afac-b08313eb92f4\"},{\"content\":{\"side\":\"TOP\"},\"type\":\"ConnectorPlacement.EquallySpacedRectSide\",\"uuid\":\"0a99e400-62af-4ce6-9b2a-3ec4b8645f60\"}]},\"type\":\"ConnectorPlacement.EquallySpacedConnector\",\"uuid\":\"ada0285e-d286-47a3-bd64-ce4f3c6c3017\"}],\"packageUris\":[\"http://schema.mathworks.com/mf0/Connector/R2020b\"],\"version\":\"1.0\"}"
  Make decision : Subsystem
      settings: PortSchema="{\"entries\":[{\"content\":{\"headerSize\":26,\"margin\":15,\"minimumSpacing\":25,\"sides\":[{\"content\":{\"connectorIds\":[\"In1\"]},\"type\":\"ConnectorPlacement.EquallySpacedRectSide\",\"uuid\":\"8049ad02-19ac-4f14-9b36-a42a8615a652\"},{\"content\":{\"connectorIds\":[\"Out1\"],\"side\":\"RIGHT\"},\"type\":\"ConnectorPlacement.EquallySpacedRectSide\",\"uuid\":\"a3e2e02d-3567-418c-afac-b08313eb92f4\"},{\"content\":{\"side\":\"TOP\"},\"type\":\"ConnectorPlacement.EquallySpacedRectSide\",\"uuid\":\"0a99e400-62af-4ce6-9b2a-3ec4b8645f60\"}]},\"type\":\"ConnectorPlacement.EquallySpacedConnector\",\"uuid\":\"ada0285e-d286-47a3-bd64-ce4f3c6c3017\"}],\"packageUris\":[\"http://schema.mathworks.com/mf0/Connector/R2020b\"],\"version\":\"1.0\"}"
  "Monitor Temperature " : Subsystem
      settings: PortSchema="{\"entries\":[{\"content\":{\"headerSize\":26,\"margin\":15,\"minimumSpacing\":25,\"sides\":[{\"content\":{\"connectorIds\":[\"In2\"]},\"type\":\"ConnectorPlacement.EquallySpacedRectSide\",\"uuid\":\"8049ad02-19ac-4f14-9b36-a42a8615a652\"},{\"content\":{\"connectorIds\":[\"Out1\",\"Out2\"],\"side\":\"RIGHT\"},\"type\":\"ConnectorPlacement.EquallySpacedRectSide\",\"uuid\":\"a3e2e02d-3567-418c-afac-b08313eb92f4\"},{\"content\":{\"side\":\"TOP\"},\"type\":\"ConnectorPlacement.EquallySpacedRectSide\",\"uuid\":\"0a99e400-62af-4ce6-9b2a-3ec4b8645f60\"},{\"content\":{\"connectorIds\":[\"In1\"],\"side\":\"BOTTOM\"},\"type\":\"ConnectorPlacement.EquallySpacedRectSide\",\"uuid\":\"3dac5849-8858-4d39-ad28-a0a278f58204\"}]},\"type\":\"ConnectorPlacement.EquallySpacedConnector\",\"uuid\":\"ada0285e-d286-47a3-bd64-ce4f3c6c3017\"}],\"packageUris\":[\"http://schema.mathworks.com/mf0/Connector/R2020b\"],\"version\":\"1.0\"}"
  Process data : Subsystem
      settings: PortSchema="{\"entries\":[{\"content\":{\"headerSize\":26,\"margin\":15,\"minimumSpacing\":25,\"sides\":[{\"content\":{\"connectorIds\":[\"In1\"]},\"type\":\"ConnectorPlacement.EquallySpacedRectSide\",\"uuid\":\"8049ad02-19ac-4f14-9b36-a42a8615a652\"},{\"content\":{\"connectorIds\":[\"Out1\"],\"side\":\"RIGHT\"},\"type\":\"ConnectorPlacement.EquallySpacedRectSide\",\"uuid\":\"a3e2e02d-3567-418c-afac-b08313eb92f4\"},{\"content\":{\"side\":\"TOP\"},\"type\":\"ConnectorPlacement.EquallySpacedRectSide\",\"uuid\":\"0a99e400-62af-4ce6-9b2a-3ec4b8645f60\"}]},\"type\":\"ConnectorPlacement.EquallySpacedConnector\",\"uuid\":\"ada0285e-d286-47a3-bd64-ce4f3c6c3017\"}],\"packageUris\":[\"http://schema.mathworks.com/mf0/Connector/R2020b\"],\"version\":\"1.0\"}"
  Receive Reed Sensor Signal : Subsystem
      settings: PortSchema="{\"entries\":[{\"content\":{\"headerSize\":26,\"margin\":15,\"minimumSpacing\":25,\"sides\":[{\"content\":{\"connectorIds\":[\"In1\",\"In2\"]},\"type\":\"ConnectorPlacement.EquallySpacedRectSide\",\"uuid\":\"8049ad02-19ac-4f14-9b36-a42a8615a652\"},{\"content\":{\"connectorIds\":[\"Out1\"],\"side\":\"RIGHT\"},\"type\":\"ConnectorPlacement.EquallySpacedRectSide\",\"uuid\":\"a3e2e02d-3567-418c-afac-b08313eb92f4\"},{\"content\":{\"side\":\"TOP\"},\"type\":\"ConnectorPlacement.EquallySpacedRectSide\",\"uuid\":\"0a99e400-62af-4ce6-9b2a-3ec4b8645f60\"}]},\"type\":\"ConnectorPlacement.EquallySpacedConnector\",\"uuid\":\"ada0285e-d286-47a3-bd64-ce4f3c6c3017\"}],\"packageUris\":[\"http://schema.mathworks.com/mf0/Connector/R2020b\"],\"version\":\"1.0\"}"
  Reduce heat : Subsystem
      settings: PortSchema="{\"entries\":[{\"content\":{\"headerSize\":26,\"margin\":15,\"minimumSpacing\":25,\"sides\":[{\"content\":{\"connectorIds\":[\"In1\"]},\"type\":\"ConnectorPlacement.EquallySpacedRectSide\",\"uuid\":\"15cbe73a-aa7b-4e66-99e8-9ab589852f2b\"},{\"content\":{\"connectorIds\":[\"Out1\"],\"side\":\"RIGHT\"},\"type\":\"ConnectorPlacement.EquallySpacedRectSide\",\"uuid\":\"676971b7-a4e3-4ea7-bcd5-348ec04a1330\"},{\"content\":{\"side\":\"TOP\"},\"type\":\"ConnectorPlacement.EquallySpacedRectSide\",\"uuid\":\"3b4cc1d2-9a88-4462-b6af-6f5c3eca2f48\"}]},\"type\":\"ConnectorPlacement.EquallySpacedConnector\",\"uuid\":\"57fb7b5e-4276-4ca9-baa4-5efca71cbc7f\"}],\"packageUris\":[\"http://schema.mathworks.com/mf0/Connector/R2020b\"],\"version\":\"1.0\"}"
  Regulate cooler : Subsystem
      settings: PortSchema="{\"entries\":[{\"content\":{\"headerSize\":26,\"margin\":15,\"minimumSpacing\":25,\"sides\":[{\"content\":{\"connectorIds\":[\"In2\"]},\"type\":\"ConnectorPlacement.EquallySpacedRectSide\",\"uuid\":\"8049ad02-19ac-4f14-9b36-a42a8615a652\"},{\"content\":{\"connectorIds\":[\"Out2\"],\"side\":\"RIGHT\"},\"type\":\"ConnectorPlacement.EquallySpacedRectSide\",\"uuid\":\"a3e2e02d-3567-418c-afac-b08313eb92f4\"},{\"content\":{\"side\":\"TOP\"},\"type\":\"ConnectorPlacement.EquallySpacedRectSide\",\"uuid\":\"0a99e400-62af-4ce6-9b2a-3ec4b8645f60\"},{\"content\":{\"connectorIds\":[\"In1\",\"Out1\"],\"side\":\"BOTTOM\"},\"type\":\"ConnectorPlacement.EquallySpacedRectSide\",\"uuid\":\"30a4d8a9-3afc-408b-9e93-eed6c6d8532c\"}]},\"type\":\"ConnectorPlacement.EquallySpacedConnector\",\"uuid\":\"ada0285e-d286-47a3-bd64-ce4f3c6c3017\"}],\"packageUris\":[\"http://schema.mathworks.com/mf0/Connector/R2020b\"],\"version\":\"1.0\"}"
  Trigger Cooling Mechanism : Subsystem
      settings: PortSchema="{\"entries\":[{\"content\":{\"headerSize\":26,\"margin\":15,\"minimumSpacing\":25,\"sides\":[{\"content\":{\"connectorIds\":[\"In2\"]},\"type\":\"ConnectorPlacement.EquallySpacedRectSide\",\"uuid\":\"8049ad02-19ac-4f14-9b36-a42a8615a652\"},{\"content\":{\"connectorIds\":[\"Out1\"],\"side\":\"RIGHT\"},\"type\":\"ConnectorPlacement.EquallySpacedRectSide\",\"uuid\":\"a3e2e02d-3567-418c-afac-b08313eb92f4\"},{\"content\":{\"side\":\"TOP\"},\"type\":\"ConnectorPlacement.EquallySpacedRectSide\",\"uuid\":\"0a99e400-62af-4ce6-9b2a-3ec4b8645f60\"},{\"content\":{\"connectorIds\":[\"In1\"],\"side\":\"BOTTOM\"},\"type\":\"ConnectorPlacement.EquallySpacedRectSide\",\"uuid\":\"e61c6aa8-48fc-4240-a4f5-0871506c3ba2\"}]},\"type\":\"ConnectorPlacement.EquallySpacedConnector\",\"uuid\":\"ada0285e-d286-47a3-bd64-ce4f3c6c3017\"}],\"packageUris\":[\"http://schema.mathworks.com/mf0/Connector/R2020b\"],\"version\":\"1.0\"}"
  Bus Element Out1 : Outport  PortName=Reed data
  Bus Element Out2 : Outport  Port=2  PortName=TemperatureIN
  wires:
  Bus Element In1/1 -> Receive Reed Sensor Signal/1(Power)
  Receive Reed Sensor Signal/1(Reed_Data) -> Detect door status/1(Reed_data)
  Detect magnetic field/1(Magnetize) -> Receive Reed Sensor Signal/2(Magnetize)
  Bus Element In3/1 -> "Monitor Temperature "/2(Power)
  "Monitor Temperature "/1(Temperature_data) -> Acquisition data/1(Temperature_data)
  Communicate status/1(Reed data) -> Bus Element Out1/1
  Detect door status/2(status_close) -> Communicate status/2(status_close)
  Detect door status/1(Status_open) -> Communicate status/1(Status_open)
  Acquisition data/1(Raw_Data) -> Process data/1(Raw_Data)
  Process data/1(Processed_Data) -> Regulate cooler/2(Processed_Data)
  Make decision/1(Alert_signal) -> Trigger Cooling Mechanism/2(Alert_signal)
  Regulate cooler/2(Cooler data) -> Make decision/1(Cooler data)
  Trigger Cooling Mechanism/1(voltage2) -> Activate Fans/1(voltage2)
  Bus Element In2/1 -> "Monitor Temperature "/1(TemperatureOUT)
  Reduce heat/1(TemperatureIN) -> Bus Element Out2/1
  "Monitor Temperature "/2(voltage) -> Regulate cooler/1(voltage)
  Regulate cooler/1(voltage1) -> Trigger Cooling Mechanism/1(voltage1)
  Activate Fans/1(fans energy) -> Reduce heat/1(fans energy)

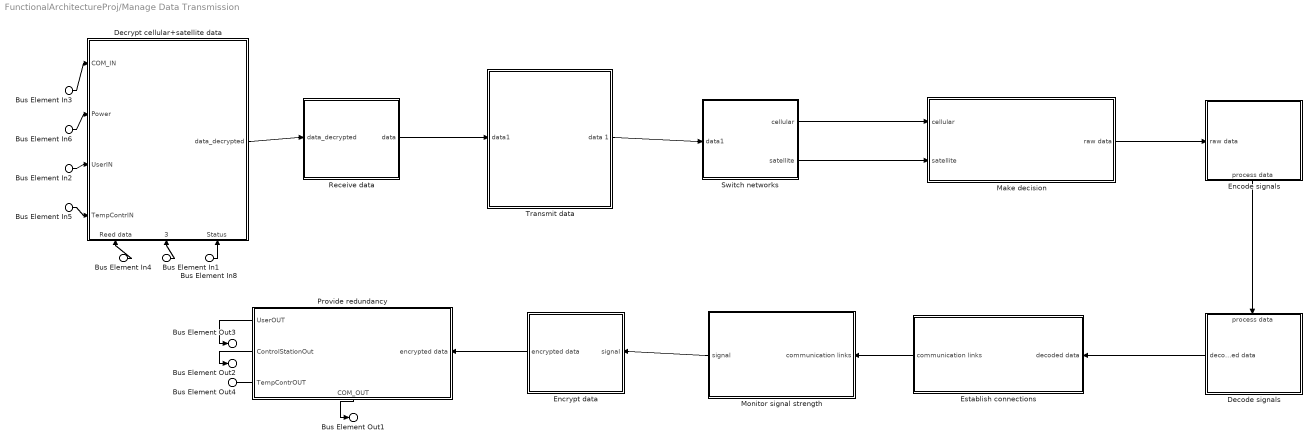
== system FunctionalArchitectureProj/Manage Data Transmission  ==
  Bus Element In8 : Inport  PortName=Status
  Bus Element In6 : Inport  Port=2  PortName=Power
  Bus Element In3 : Inport  Port=3  PortName=COM_IN
  Bus Element In1 : Inport  Port=4  PortName=ControlStationIN
  Bus Element In2 : Inport  Port=5  PortName=UserIN
  Bus Element In4 : Inport  Port=6  PortName=Reed data
  Bus Element In5 : Inport  Port=7  PortName=TempContrIN
  Decode signals : Subsystem
      settings: PortSchema="{\"entries\":[{\"content\":{\"headerSize\":26,\"margin\":15,\"minimumSpacing\":25,\"sides\":[{\"content\":{\"connectorIds\":[\"Out1\"]},\"type\":\"ConnectorPlacement.EquallySpacedRectSide\",\"uuid\":\"15cbe73a-aa7b-4e66-99e8-9ab589852f2b\"},{\"content\":{\"side\":\"RIGHT\"},\"type\":\"ConnectorPlacement.EquallySpacedRectSide\",\"uuid\":\"676971b7-a4e3-4ea7-bcd5-348ec04a1330\"},{\"content\":{\"connectorIds\":[\"In1\"],\"side\":\"TOP\"},\"type\":\"ConnectorPlacement.EquallySpacedRectSide\",\"uuid\":\"3b4cc1d2-9a88-4462-b6af-6f5c3eca2f48\"}]},\"type\":\"ConnectorPlacement.EquallySpacedConnector\",\"uuid\":\"57fb7b5e-4276-4ca9-baa4-5efca71cbc7f\"}],\"packageUris\":[\"http://schema.mathworks.com/mf0/Connector/R2020b\"],\"version\":\"1.0\"}"
  Decrypt cellular+satellite data : Subsystem
      settings: PortSchema="{\"entries\":[{\"content\":{\"headerSize\":26,\"margin\":15,\"minimumSpacing\":25,\"sides\":[{\"content\":{\"connectorIds\":[\"In2\",\"In6\",\"In7\",\"In5\"]},\"type\":\"ConnectorPlacement.EquallySpacedRectSide\",\"uuid\":\"15cbe73a-aa7b-4e66-99e8-9ab589852f2b\"},{\"content\":{\"connectorIds\":[\"Out1\"],\"side\":\"RIGHT\"},\"type\":\"ConnectorPlacement.EquallySpacedRectSide\",\"uuid\":\"676971b7-a4e3-4ea7-bcd5-348ec04a1330\"},{\"content\":{\"side\":\"TOP\"},\"type\":\"ConnectorPlacement.EquallySpacedRectSide\",\"uuid\":\"3b4cc1d2-9a88-4462-b6af-6f5c3eca2f48\"},{\"content\":{\"connectorIds\":[\"In1\",\"In3\",\"In4\"],\"side\":\"BOTTOM\"},\"type\":\"ConnectorPlacement.EquallySpacedRectSide\",\"uuid\":\"5b101011-cf4a-452e-b443-25ed6938d836\"}]},\"type\":\"ConnectorPlacement.EquallySpacedConnector\",\"uuid\":\"57fb7b5e-4276-4ca9-baa4-5efca71cbc7f\"}],\"packageUris\":[\"http://schema.mathworks.com/mf0/Connector/R2020b\"],\"version\":\"1.0\"}"
  Encode signals : Subsystem
      settings: PortSchema="{\"entries\":[{\"content\":{\"headerSize\":26,\"margin\":15,\"minimumSpacing\":25,\"sides\":[{\"content\":{\"connectorIds\":[\"In1\"]},\"type\":\"ConnectorPlacement.EquallySpacedRectSide\",\"uuid\":\"15cbe73a-aa7b-4e66-99e8-9ab589852f2b\"},{\"content\":{\"side\":\"RIGHT\"},\"type\":\"ConnectorPlacement.EquallySpacedRectSide\",\"uuid\":\"676971b7-a4e3-4ea7-bcd5-348ec04a1330\"},{\"content\":{\"side\":\"TOP\"},\"type\":\"ConnectorPlacement.EquallySpacedRectSide\",\"uuid\":\"3b4cc1d2-9a88-4462-b6af-6f5c3eca2f48\"},{\"content\":{\"connectorIds\":[\"Out1\"],\"side\":\"BOTTOM\"},\"type\":\"ConnectorPlacement.EquallySpacedRectSide\",\"uuid\":\"10a2b569-cb90-4db8-a835-178104b57e5b\"}]},\"type\":\"ConnectorPlacement.EquallySpacedConnector\",\"uuid\":\"57fb7b5e-4276-4ca9-baa4-5efca71cbc7f\"}],\"packageUris\":[\"http://schema.mathworks.com/mf0/Connector/R2020b\"],\"version\":\"1.0\"}"
  Encrypt data : Subsystem
      settings: PortSchema="{\"entries\":[{\"content\":{\"headerSize\":26,\"margin\":15,\"minimumSpacing\":25,\"sides\":[{\"content\":{\"connectorIds\":[\"Out1\"]},\"type\":\"ConnectorPlacement.EquallySpacedRectSide\",\"uuid\":\"15cbe73a-aa7b-4e66-99e8-9ab589852f2b\"},{\"content\":{\"connectorIds\":[\"In1\"],\"side\":\"RIGHT\"},\"type\":\"ConnectorPlacement.EquallySpacedRectSide\",\"uuid\":\"676971b7-a4e3-4ea7-bcd5-348ec04a1330\"},{\"content\":{\"side\":\"TOP\"},\"type\":\"ConnectorPlacement.EquallySpacedRectSide\",\"uuid\":\"3b4cc1d2-9a88-4462-b6af-6f5c3eca2f48\"}]},\"type\":\"ConnectorPlacement.EquallySpacedConnector\",\"uuid\":\"57fb7b5e-4276-4ca9-baa4-5efca71cbc7f\"}],\"packageUris\":[\"http://schema.mathworks.com/mf0/Connector/R2020b\"],\"version\":\"1.0\"}"
  Establish connections : Subsystem
      settings: PortSchema="{\"entries\":[{\"content\":{\"headerSize\":26,\"margin\":15,\"minimumSpacing\":25,\"sides\":[{\"content\":{\"connectorIds\":[\"Out1\"]},\"type\":\"ConnectorPlacement.EquallySpacedRectSide\",\"uuid\":\"15cbe73a-aa7b-4e66-99e8-9ab589852f2b\"},{\"content\":{\"connectorIds\":[\"In1\"],\"side\":\"RIGHT\"},\"type\":\"ConnectorPlacement.EquallySpacedRectSide\",\"uuid\":\"676971b7-a4e3-4ea7-bcd5-348ec04a1330\"},{\"content\":{\"side\":\"TOP\"},\"type\":\"ConnectorPlacement.EquallySpacedRectSide\",\"uuid\":\"3b4cc1d2-9a88-4462-b6af-6f5c3eca2f48\"}]},\"type\":\"ConnectorPlacement.EquallySpacedConnector\",\"uuid\":\"57fb7b5e-4276-4ca9-baa4-5efca71cbc7f\"}],\"packageUris\":[\"http://schema.mathworks.com/mf0/Connector/R2020b\"],\"version\":\"1.0\"}"
  Make decision : Subsystem
      settings: PortSchema="{\"entries\":[{\"content\":{\"headerSize\":26,\"margin\":15,\"minimumSpacing\":25,\"sides\":[{\"content\":{\"connectorIds\":[\"In2\",\"In1\"]},\"type\":\"ConnectorPlacement.EquallySpacedRectSide\",\"uuid\":\"15cbe73a-aa7b-4e66-99e8-9ab589852f2b\"},{\"content\":{\"connectorIds\":[\"Out1\"],\"side\":\"RIGHT\"},\"type\":\"ConnectorPlacement.EquallySpacedRectSide\",\"uuid\":\"676971b7-a4e3-4ea7-bcd5-348ec04a1330\"},{\"content\":{\"side\":\"TOP\"},\"type\":\"ConnectorPlacement.EquallySpacedRectSide\",\"uuid\":\"3b4cc1d2-9a88-4462-b6af-6f5c3eca2f48\"},{\"content\":{\"side\":\"BOTTOM\"},\"type\":\"ConnectorPlacement.EquallySpacedRectSide\",\"uuid\":\"b5503ab4-a703-4e48-a0aa-3feba21ce30b\"}]},\"type\":\"ConnectorPlacement.EquallySpacedConnector\",\"uuid\":\"57fb7b5e-4276-4ca9-baa4-5efca71cbc7f\"}],\"packageUris\":[\"http://schema.mathworks.com/mf0/Connector/R2020b\"],\"version\":\"1.0\"}"
  Monitor signal strength : Subsystem
      settings: PortSchema="{\"entries\":[{\"content\":{\"headerSize\":26,\"margin\":15,\"minimumSpacing\":25,\"sides\":[{\"content\":{\"connectorIds\":[\"Out1\"]},\"type\":\"ConnectorPlacement.EquallySpacedRectSide\",\"uuid\":\"15cbe73a-aa7b-4e66-99e8-9ab589852f2b\"},{\"content\":{\"connectorIds\":[\"In1\"],\"side\":\"RIGHT\"},\"type\":\"ConnectorPlacement.EquallySpacedRectSide\",\"uuid\":\"676971b7-a4e3-4ea7-bcd5-348ec04a1330\"},{\"content\":{\"side\":\"TOP\"},\"type\":\"ConnectorPlacement.EquallySpacedRectSide\",\"uuid\":\"3b4cc1d2-9a88-4462-b6af-6f5c3eca2f48\"}]},\"type\":\"ConnectorPlacement.EquallySpacedConnector\",\"uuid\":\"57fb7b5e-4276-4ca9-baa4-5efca71cbc7f\"}],\"packageUris\":[\"http://schema.mathworks.com/mf0/Connector/R2020b\"],\"version\":\"1.0\"}"
  Provide redundancy : Subsystem
      settings: PortSchema="{\"entries\":[{\"content\":{\"headerSize\":26,\"margin\":15,\"minimumSpacing\":25,\"sides\":[{\"content\":{\"connectorIds\":[\"Out2\",\"Out3\",\"Out4\"]},\"type\":\"ConnectorPlacement.EquallySpacedRectSide\",\"uuid\":\"15cbe73a-aa7b-4e66-99e8-9ab589852f2b\"},{\"content\":{\"connectorIds\":[\"In1\"],\"side\":\"RIGHT\"},\"type\":\"ConnectorPlacement.EquallySpacedRectSide\",\"uuid\":\"676971b7-a4e3-4ea7-bcd5-348ec04a1330\"},{\"content\":{\"side\":\"TOP\"},\"type\":\"ConnectorPlacement.EquallySpacedRectSide\",\"uuid\":\"3b4cc1d2-9a88-4462-b6af-6f5c3eca2f48\"},{\"content\":{\"connectorIds\":[\"Out1\"],\"side\":\"BOTTOM\"},\"type\":\"ConnectorPlacement.EquallySpacedRectSide\",\"uuid\":\"b46eefc0-683f-4c29-9b04-b4928f92bbaa\"}]},\"type\":\"ConnectorPlacement.EquallySpacedConnector\",\"uuid\":\"57fb7b5e-4276-4ca9-baa4-5efca71cbc7f\"}],\"packageUris\":[\"http://schema.mathworks.com/mf0/Connector/R2020b\"],\"version\":\"1.0\"}"
  Receive data : Subsystem
      settings: PortSchema="{\"entries\":[{\"content\":{\"headerSize\":26,\"margin\":15,\"minimumSpacing\":25,\"sides\":[{\"content\":{\"connectorIds\":[\"In1\"]},\"type\":\"ConnectorPlacement.EquallySpacedRectSide\",\"uuid\":\"15cbe73a-aa7b-4e66-99e8-9ab589852f2b\"},{\"content\":{\"connectorIds\":[\"Out1\"],\"side\":\"RIGHT\"},\"type\":\"ConnectorPlacement.EquallySpacedRectSide\",\"uuid\":\"676971b7-a4e3-4ea7-bcd5-348ec04a1330\"},{\"content\":{\"side\":\"TOP\"},\"type\":\"ConnectorPlacement.EquallySpacedRectSide\",\"uuid\":\"3b4cc1d2-9a88-4462-b6af-6f5c3eca2f48\"}]},\"type\":\"ConnectorPlacement.EquallySpacedConnector\",\"uuid\":\"57fb7b5e-4276-4ca9-baa4-5efca71cbc7f\"}],\"packageUris\":[\"http://schema.mathworks.com/mf0/Connector/R2020b\"],\"version\":\"1.0\"}"
  Switch networks : Subsystem
      settings: PortSchema="{\"entries\":[{\"content\":{\"headerSize\":26,\"margin\":15,\"minimumSpacing\":25,\"sides\":[{\"content\":{\"connectorIds\":[\"In1\"]},\"type\":\"ConnectorPlacement.EquallySpacedRectSide\",\"uuid\":\"15cbe73a-aa7b-4e66-99e8-9ab589852f2b\"},{\"content\":{\"connectorIds\":[\"Out1\",\"Out2\"],\"side\":\"RIGHT\"},\"type\":\"ConnectorPlacement.EquallySpacedRectSide\",\"uuid\":\"676971b7-a4e3-4ea7-bcd5-348ec04a1330\"},{\"content\":{\"side\":\"TOP\"},\"type\":\"ConnectorPlacement.EquallySpacedRectSide\",\"uuid\":\"3b4cc1d2-9a88-4462-b6af-6f5c3eca2f48\"}]},\"type\":\"ConnectorPlacement.EquallySpacedConnector\",\"uuid\":\"57fb7b5e-4276-4ca9-baa4-5efca71cbc7f\"}],\"packageUris\":[\"http://schema.mathworks.com/mf0/Connector/R2020b\"],\"version\":\"1.0\"}"
  Transmit data : Subsystem
      settings: PortSchema="{\"entries\":[{\"content\":{\"headerSize\":26,\"margin\":15,\"minimumSpacing\":25,\"sides\":[{\"content\":{\"connectorIds\":[\"In1\"]},\"type\":\"ConnectorPlacement.EquallySpacedRectSide\",\"uuid\":\"15cbe73a-aa7b-4e66-99e8-9ab589852f2b\"},{\"content\":{\"connectorIds\":[\"Out1\"],\"side\":\"RIGHT\"},\"type\":\"ConnectorPlacement.EquallySpacedRectSide\",\"uuid\":\"676971b7-a4e3-4ea7-bcd5-348ec04a1330\"},{\"content\":{\"side\":\"TOP\"},\"type\":\"ConnectorPlacement.EquallySpacedRectSide\",\"uuid\":\"3b4cc1d2-9a88-4462-b6af-6f5c3eca2f48\"},{\"content\":{\"side\":\"BOTTOM\"},\"type\":\"ConnectorPlacement.EquallySpacedRectSide\",\"uuid\":\"528ebee6-e2e8-41b4-9a07-d475b7f38321\"}]},\"type\":\"ConnectorPlacement.EquallySpacedConnector\",\"uuid\":\"57fb7b5e-4276-4ca9-baa4-5efca71cbc7f\"}],\"packageUris\":[\"http://schema.mathworks.com/mf0/Connector/R2020b\"],\"version\":\"1.0\"}"
  Bus Element Out1 : Outport  PortName=COM_OUT
  Bus Element Out3 : Outport  Port=2  PortName=UserOUT
  Bus Element Out2 : Outport  Port=3  PortName=ControlStationOut
  Bus Element Out4 : Outport  Port=4  PortName=TempContrOUT
  wires:
  Switch networks/1(cellular) -> Make decision/2(cellular)
  Make decision/1(raw data) -> Encode signals/1(raw data)
  Bus Element In6/1 -> Decrypt cellular+satellite data/6(Power)
  Bus Element In2/1 -> Decrypt cellular+satellite data/7(UserIN)
  Bus Element In8/1 -> Decrypt cellular+satellite data/4(Status)
  Bus Element In1/1 -> Decrypt cellular+satellite data/3(ControlStationIN)
  Bus Element In3/1 -> Decrypt cellular+satellite data/2(COM_IN)
  Bus Element In5/1 -> Decrypt cellular+satellite data/5(TempContrIN)
  Bus Element In4/1 -> Decrypt cellular+satellite data/1(Reed data)
  Switch networks/2(satellite) -> Make decision/1(satellite)
  Encode signals/1(process data) -> Decode signals/1(process data)
  Decode signals/1(decoded data) -> Establish connections/1(decoded data)
  Establish connections/1(communication links) -> Monitor signal strength/1(communication links)
  Monitor signal strength/1(signal) -> Encrypt data/1(signal)
  Encrypt data/1(encrypted data) -> Provide redundancy/1(encrypted data)
  Provide redundancy/4(TempContrOUT) -> Bus Element Out4/1
  Provide redundancy/3(ControlStationOut) -> Bus Element Out2/1
  Provide redundancy/2(UserOUT) -> Bus Element Out3/1
  Provide redundancy/1(COM_OUT) -> Bus Element Out1/1
  Decrypt cellular+satellite data/1(data_decrypted) -> Receive data/1(data_decrypted)
  Transmit data/1(data 1) -> Switch networks/1(data1)
  Receive data/1(data) -> Transmit data/1(data1)
